simulink model "motor_position_control"  (R2025b)
settings: Solver=VariableStepAuto  StartTime=0.0  StopTime=10.0  RelTol=1e-3
values from neighbouring files (symbols this model uses):
  Kp = 5    [inverted_pendulum_testing.m]    (also in motor_response_multiple.m = ii; motor_response_single.m = 8)
undefined symbols (not defined in the file or in its folder): b, J, K, L, R
settings Model: Creator=REARDONNM24  LastModifiedBy=REARDONNM24

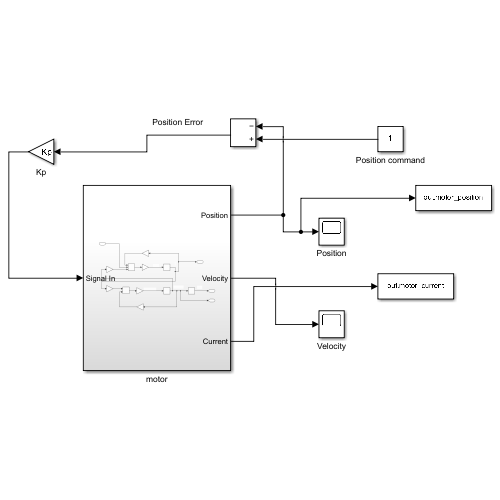
[thumbnail: Simulink's stored preview of the top-level diagram]
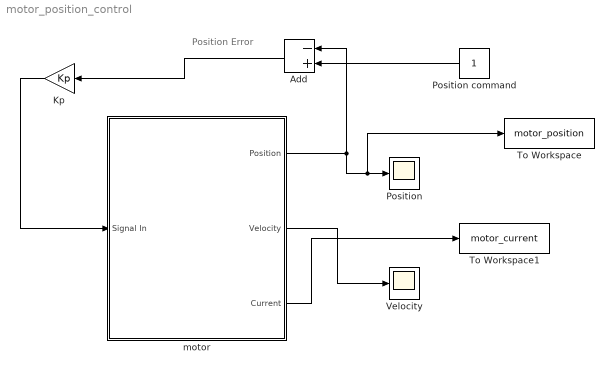
== system motor_position_control ==
  note: Position Error
  Add : Sum  Inputs=-+
  Kp : Gain  Gain=Kp
  Position : Scope
      settings: ActiveDisplayYMinimum=0.90254200315002775  ActiveDisplayYMaximum=1.0689345783117008
  Position command : Constant
  To Workspace : ToWorkspace  VariableName=motor_position  SaveFormat=Timeseries  SampleTime=-1
  To Workspace1 : ToWorkspace  VariableName=motor_current  SaveFormat=Timeseries  SampleTime=-1
  Velocity : Scope
      settings: ActiveDisplayYMinimum=174.41543511722466  ActiveDisplayYMaximum=4357.1108128089754
  motor : Subsystem
  wires:
  motor/1(Position) -> To Workspace/1, Position/1, Add/1
  motor/2(Velocity) -> Velocity/1
  Add/1 -> Kp/1
  Kp/1 -> motor/1(Signal In)
  Position command/1 -> Add/2
  motor/3(Current) -> To Workspace1/1

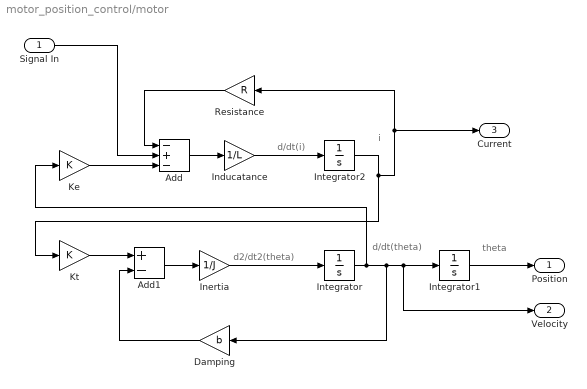
== system motor_position_control/motor ==
  note: i
  note: d/dt(i)
  note: theta
  note: d/dt(theta)
  note: d2/dt2(theta)
  Signal In : Inport
  Add : Sum  Inputs=-+-
  Add1 : Sum  Inputs=+-
  Damping : Gain  Gain=b
  Inducatance : Gain  Gain=1/L
  Inertia : Gain  Gain=1/J
  Integrator : Integrator
  Integrator1 : Integrator
  Integrator2 : Integrator
  Ke : Gain  Gain=K
  Kt : Gain  Gain=K
  Resistance : Gain  Gain=R
  Position : Outport
  Velocity : Outport  Port=2
  Current : Outport  Port=3
  wires:
  Signal In/1 -> Add/2
  Resistance/1 -> Add/1
  Inertia/1 -> Integrator/1
  Integrator/1 -> Ke/1, Damping/1, Velocity/1, Integrator1/1
  Integrator2/1 -> Current/1, Resistance/1, Kt/1
  Damping/1 -> Add1/2
  Inducatance/1 -> Integrator2/1
  Add1/1 -> Inertia/1
  Add/1 -> Inducatance/1
  Kt/1 -> Add1/1
  Ke/1 -> Add/3
  Integrator1/1 -> Position/1
